simulink model "non_linear_h1_h2"  (R2024b)
settings: Solver=VariableStepAuto  StartTime=0.0  StopTime=100  RelTol=1e-8
settings Model: Creator=apm3  LastModifiedBy=baley

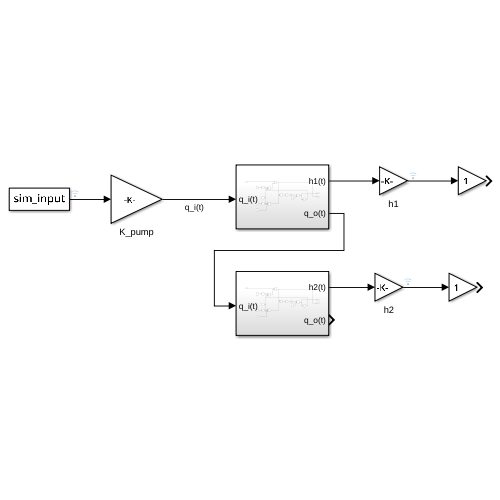
[thumbnail: Simulink's stored preview of the top-level diagram]
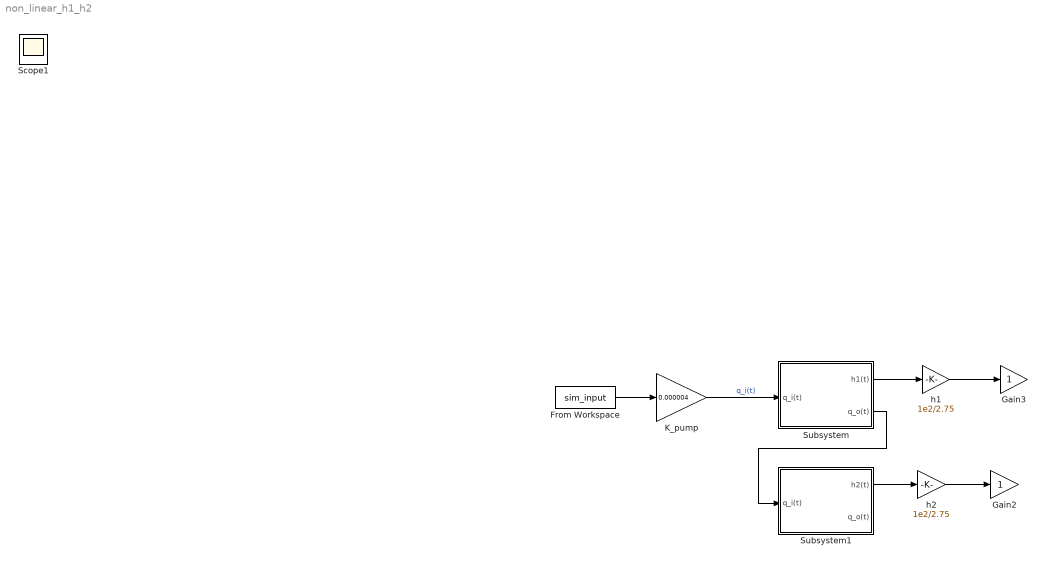
== system non_linear_h1_h2 ==
  From Workspace : FromWorkspace  VariableName=sim_input
  Gain2 : Gain
  Gain3 : Gain
  K_pump : Gain  Gain=0.000004
  Subsystem : Subsystem
  Subsystem1 : Subsystem
  h1 : Gain  Gain=1e2/2.75
  h2 : Gain  Gain=1e2/2.75
  Scope1 : Scope
  wires:
  From Workspace/1 -> K_pump/1
  K_pump/1 -> Subsystem/1(q_i(t))  "q_i(t)"
  Subsystem/2(q_o(t)) -> Subsystem1/1(q_i(t))
  Subsystem/1(h1(t)) -> h1/1
  Subsystem1/1(h2(t)) -> h2/1
  h2/1 -> Gain2/1
  h1/1 -> Gain3/1

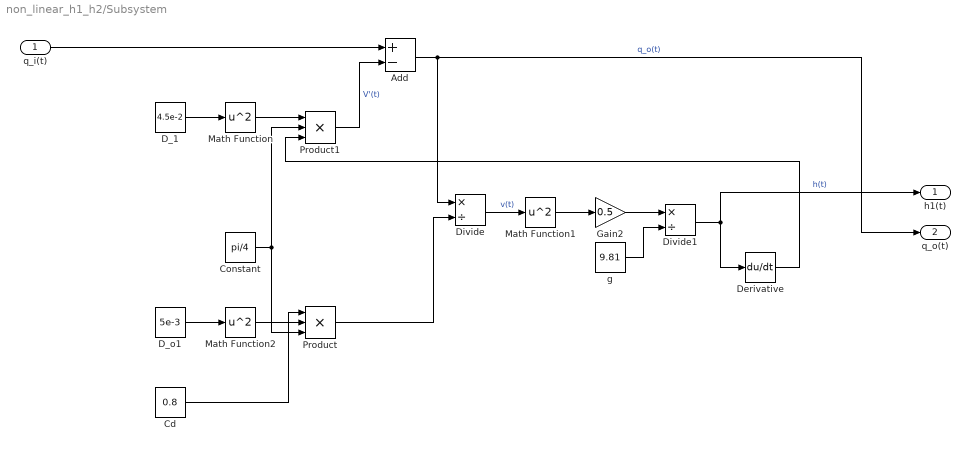
== system non_linear_h1_h2/Subsystem ==
  q_i(t) : Inport
  Add : Sum  Inputs=+-
  Cd : Constant  Value=0.8
  Constant : Constant  Value=pi/4
  D_1 : Constant  Value=4.5e-2
  D_o1 : Constant  Value=5e-3
  Derivative : Derivative
  Divide : Product  Inputs=*/
  Divide1 : Product  Inputs=*/
  Gain2 : Gain  Gain=0.5
  Math Function : Math  Operator=square
  Math Function1 : Math  Operator=square
  Math Function2 : Math  Operator=square
  Product : Product  Inputs=3
  Product1 : Product  Inputs=3
  g : Constant  Value=9.81
  h1(t) : Outport
  q_o(t) : Outport  Port=2
  wires:
  Cd/1 -> Product/1
  Constant/1 -> Product/3, Product1/2
  D_1/1 -> Math Function/1
  g/1 -> Divide1/2
  Math Function1/1 -> Gain2/1
  D_o1/1 -> Math Function2/1
  Add/1 -> q_o(t)/1, Divide/1  "q_o(t)"
  Math Function2/1 -> Product/2
  Math Function/1 -> Product1/1
  q_i(t)/1 -> Add/1
  Divide1/1 -> h1(t)/1, Derivative/1  "h(t)"
  Product/1 -> Divide/2
  Product1/1 -> Add/2  "V'(t)"
  Gain2/1 -> Divide1/1
  Divide/1 -> Math Function1/1  "v(t)"
  Derivative/1 -> Product1/3

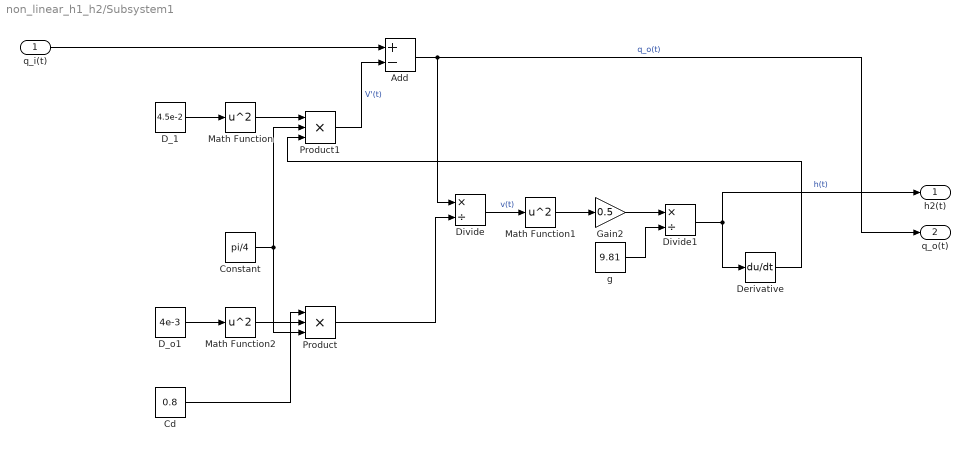
== system non_linear_h1_h2/Subsystem1 ==
  q_i(t) : Inport
  Add : Sum  Inputs=+-
  Cd : Constant  Value=0.8
  Constant : Constant  Value=pi/4
  D_1 : Constant  Value=4.5e-2
  D_o1 : Constant  Value=4e-3
  Derivative : Derivative
  Divide : Product  Inputs=*/
  Divide1 : Product  Inputs=*/
  Gain2 : Gain  Gain=0.5
  Math Function : Math  Operator=square
  Math Function1 : Math  Operator=square
  Math Function2 : Math  Operator=square
  Product : Product  Inputs=3
  Product1 : Product  Inputs=3
  g : Constant  Value=9.81
  h2(t) : Outport
  q_o(t) : Outport  Port=2
  wires:
  Cd/1 -> Product/1
  Constant/1 -> Product/3, Product1/2
  D_1/1 -> Math Function/1
  g/1 -> Divide1/2
  Math Function1/1 -> Gain2/1
  D_o1/1 -> Math Function2/1
  Add/1 -> q_o(t)/1, Divide/1  "q_o(t)"
  Math Function2/1 -> Product/2
  Math Function/1 -> Product1/1
  q_i(t)/1 -> Add/1
  Divide1/1 -> h2(t)/1, Derivative/1  "h(t)"
  Product/1 -> Divide/2
  Product1/1 -> Add/2  "V'(t)"
  Gain2/1 -> Divide1/1
  Divide/1 -> Math Function1/1  "v(t)"
  Derivative/1 -> Product1/3
